simulink model "main_sim_adapt_Gref_SPPH"  (Simulink 7.2)
settings: Solver=ode2  SolverMode=SingleTasking  StartTime=0.0  StopTime=tsim_max  FixedStep=dtsim  RelTol=1e-3
StopFcn:
  | %mkplt
values from neighbouring files (symbols this model uses):
  assertion_time = inf    [setup_taem_sgs_al.m]
  cosA = cos(rwyAZ_rad)    [setup_taem_sgs_al.m]
  E_rwy = E_origin + (mod(( rwyLLA(2)/constants.r2d - lon_origin )+pi,2*pi)-pi) * constants.earth_radius * cos(lat_origin)    [setup_taem_sgs_al.m]
  eow_boundary = tmp_eow(ix(1))    [setup_taem_sgs_al.m]
  N_rwy = N_origin + (mod(( rwyLLA(1)/constants.r2d - lat_origin )+pi,2*pi)-pi) * constants.earth_radius    [setup_taem_sgs_al.m]
  sinA = sin(rwyAZ_rad)    [setup_taem_sgs_al.m]
  vel = 487.2512    [doit.m]
undefined symbols (not defined in the file or in its folder): accel_cmd, aero_surf_qbar_off, aero_surf_qbar_on, Alon, att_cmd_select, att_trim_IC, att_type, att_type_numbers, B1, bb_ellipsoid, bb_params, Blon, C, CA, chi_trim_IC, Clon, command_time, compute_all_rate_cols, compute_all_vel_cols, constants, da_trim_IC, dc_L2W_IC, de_trim_IC, DiscIntNeverNeededParam, dr_trim_IC, dtsim, DZkx, DZtheta, E_trim_IC, Ed_cmd, Ed_trim_IC, fc, flag_uad, full_surf_llim, full_surf_ulim, gain_set, gain_var_struct, gam_cmd_descent, gam_cmd_preflare, gamdot_cmd_descent, gamdot_cmd_flare, gamdot_cmd_preflare, gamma_trim_IC, Gamtheta, Gamx, h_trim_IC, hd_cmd, hd_trim_IC, ideal_vel_Kb, in_exsig_vecin, in_exsig_vecout, invCB, Kb, Kxhat0, Kxnom, Kxstar, lonxm0, MACH, MACH_att_fb, MACH_att_int_IC ... (+77)
libraries: simulink x36, utility_lib x36, mach_lib x24, model_lib x15, simulink_need_slupdate x8, models x6
(part 7 of 7)

== system main_sim_adapt_Gref_SPPH/claw_main/vel_loops/B matrix comp/B matrix comp/pert_comp ==
  col : Inport  OutDataType=sfix(16)  OutScaling=2^0
  d_nom : Inport  Port=2  OutDataType=sfix(16)  OutScaling=2^0
  params : Inport  Port=3  OutDataType=sfix(16)  OutScaling=2^0
  Bus Selector : BusSelector  OutputSignals=u_ulim,u_llim
  Constant2 : Constant  Value=diag(MACH.vel_u_pert)  OutDataType=sfix(16)  OutScaling=2^0
  pick +/- pert : mach_lib/pick +//- pert  SystemSampleTime=-1  num_u=MACH.vel_num_u
  d_pert : Outport  OutDataType=sfix(16)  OutScaling=2^0
  d_div : Outport  Port=2  OutDataType=sfix(16)  OutScaling=2^0
  wires:
  pick +/- pert/2 -> d_div/1  "scalar pert value"
  d_nom/1 -> pick +/- pert/2
  pick +/- pert/1 -> d_pert/1
  col/1 -> pick +/- pert/1
  Constant2/1 -> pick +/- pert/5
  params/1 -> Bus Selector/1
  Bus Selector/1 -> pick +/- pert/3  "<u_ulim>"
  Bus Selector/2 -> pick +/- pert/4  "<u_llim>"

== system main_sim_adapt_Gref_SPPH/claw_main/vel_loops/convert accel_cmd to NED_dd_cmd/vchigam_dot cmd/polar to cart ==
  note: Note: these are actually Vground and Vslant
  scaling_info : Inport  OutDataType=sfix(16)  OutScaling=2^0
  vchigam_dot_cmd : Inport  Port=2  OutDataType=sfix(16)  OutScaling=2^0
  Bus Selector : BusSelector  OutputSignals=Rground,Rslant
  Demux : Demux  Outputs=[1 2]
  Gain1 : Gain  Gain=[1 -1]  ParameterDataType=sfix(16)  ParameterScaling=2^0  OutDataType=sfix(16)  OutScaling=2^0
  Mux : Mux  Inputs=2
  Mux1 : Mux  Inputs=2
  Product3 : Product  OutDataType=sfix(16)  OutScaling=2^0  RndMeth=Zero
  along_dd;cross_dd;vert_dd : Outport  OutDataType=sfix(16)  OutScaling=2^0
  wires:
  scaling_info/1 -> Bus Selector/1
  Mux/1 -> Gain1/1
  vchigam_dot_cmd/1 -> Demux/1
  Bus Selector/1 -> Mux/1  "<Rground>"
  Bus Selector/2 -> Mux/2  "<Rslant>"
  Gain1/1 -> Product3/2
  Demux/2 -> Product3/1
  Demux/1 -> Mux1/1
  Product3/1 -> Mux1/2
  Mux1/1 -> along_dd;cross_dd;vert_dd/1

== system main_sim_adapt_Gref_SPPH/control input (modified)/control input/form control input/select command/att cmd select ==
  cmd_bus : Inport  OutDataType=sfix(16)  OutScaling=2^0
  Bus Selector1 : BusSelector  OutputSignals=att1_cmd,att2_cmd,att3_cmd,throttle_cmd  OutputAsBus=on
  Bus Selector2 : BusSelector  OutputSignals=att_cmd
  Switch : Switch  Threshold=0.5
  use_cam_rate_cmd1 : Constant  Value=att_cmd_select  OutDataType=sfix(16)  OutScaling=2^0
  att_cmd : Outport  OutDataType=sfix(16)  OutScaling=2^0
  wires:
  Switch/1 -> att_cmd/1
  use_cam_rate_cmd1/1 -> Switch/2
  cmd_bus/1 -> Bus Selector2/1, Bus Selector1/1
  Bus Selector2/1 -> Switch/1  "<att_cmd>"
  Bus Selector1/1 -> Switch/3

== system main_sim_adapt_Gref_SPPH/control input (modified)/control input/form control input/select command/pos cmd select ==
  cmd_bus : Inport  OutDataType=sfix(16)  OutScaling=2^0
  Bus Selector1 : BusSelector  OutputSignals=N_cmd,E_cmd,att3_cmd,h_cmd  OutputAsBus=on
  Bus Selector3 : BusSelector  OutputSignals=pos_cmd,accel_submode
  Bus Selector5 : BusSelector  OutputSignals=Vd_cmd,chid_cmd,att3_cmd,gammad_cmd  OutputAsBus=on
  Bus Selector6 : BusSelector  OutputSignals=Ndd_cmd,Edd_cmd,att3_cmd,hdd_cmd  OutputAsBus=on
  Constant : Constant  Value=use_NdEdh_pos  OutDataType=sfix(16)  OutScaling=2^0
  Ground : Ground
  Multiport Switch : MultiPortSwitch  Inputs=2  zeroidx=on
  Multiport Switch1 : MultiPortSwitch  Inputs=4  zeroidx=on
  Switch : Switch  Threshold=0.5
  convert if use_Vchigam : Subsystem
  use_cam_rate_cmd1 : Constant  Value=pos_cmd_select  OutDataType=sfix(16)  OutScaling=2^0
  pos_cmd : Outport  OutDataType=sfix(16)  OutScaling=2^0
  wires:
  Multiport Switch1/1 -> Switch/3
  Bus Selector5/1 -> Multiport Switch1/4
  Bus Selector6/1 -> Multiport Switch1/3
  Ground/1 -> Multiport Switch1/5
  Multiport Switch/1 -> Multiport Switch1/2
  Bus Selector3/2 -> Multiport Switch1/1  "<accel_submode>"
  Bus Selector3/1 -> Switch/1  "<pos_cmd>"
  Switch/1 -> pos_cmd/1
  use_cam_rate_cmd1/1 -> Switch/2
  cmd_bus/1 -> Bus Selector3/1, convert if use_Vchigam/1(cmd_bus), Bus Selector5/1, Bus Selector6/1, Bus Selector1/1
  Bus Selector1/1 -> Multiport Switch/2
  convert if use_Vchigam/1(pos_cmd) -> Multiport Switch/3
  Constant/1 -> Multiport Switch/1

== system main_sim_adapt_Gref_SPPH/control input (modified)/control input/form control input/select command/rate cmd select ==
  cmd_bus : Inport  OutDataType=sfix(16)  OutScaling=2^0
  Bus Selector1 : BusSelector  OutputSignals=p_cmd,q_cmd,r_cmd,throttle_cmd  OutputAsBus=on
  Bus Selector3 : BusSelector  OutputSignals=rate_cmd  OutputAsBus=on
  Switch : Switch  Threshold=0.5
  use_cam_rate_cmd1 : Constant  Value=rate_cmd_select  OutDataType=sfix(16)  OutScaling=2^0
  rate_cmd : Outport  OutDataType=sfix(16)  OutScaling=2^0
  wires:
  Bus Selector1/1 -> Switch/3
  Bus Selector3/1 -> Switch/1
  cmd_bus/1 -> Bus Selector1/1, Bus Selector3/1
  use_cam_rate_cmd1/1 -> Switch/2
  Switch/1 -> rate_cmd/1

== system main_sim_adapt_Gref_SPPH/control input (modified)/control input/form control input/select command/vel cmd select ==
  cmd_bus : Inport  OutDataType=sfix(16)  OutScaling=2^0
  Bus Selector1 : BusSelector  OutputSignals=Vd_cmd,chid_cmd,att3_cmd,gammad_cmd  OutputAsBus=on
  Bus Selector2 : BusSelector  OutputSignals=vel_cmd,accel_submode
  Bus Selector4 : BusSelector  OutputSignals=Ndd_cmd,Edd_cmd,att3_cmd,hdd_cmd  OutputAsBus=on
  Ground : Ground
  Multiport Switch : MultiPortSwitch  Inputs=4  zeroidx=on
  Switch : Switch  Threshold=0.5
  convert if use_Vchigam : Subsystem
  use_cam_rate_cmd1 : Constant  Value=vel_cmd_select  OutDataType=sfix(16)  OutScaling=2^0
  vel_cmd : Outport  OutDataType=sfix(16)  OutScaling=2^0
  wires:
  convert if use_Vchigam/1(vel_cmd) -> Multiport Switch/2
  Multiport Switch/1 -> Switch/3
  Bus Selector1/1 -> Multiport Switch/4
  Ground/1 -> Multiport Switch/5
  Bus Selector4/1 -> Multiport Switch/3
  Bus Selector2/2 -> Multiport Switch/1  "<accel_submode>"
  Bus Selector2/1 -> Switch/1  "<vel_cmd>"
  cmd_bus/1 -> convert if use_Vchigam/1(cmd_bus), Bus Selector1/1, Bus Selector4/1, Bus Selector2/1
  use_cam_rate_cmd1/1 -> Switch/2
  Switch/1 -> vel_cmd/1

== system main_sim_adapt_Gref_SPPH/control input (modified)/control input/generate commands/pos cmd generator/circle pos cmd ==
  cmd_bus : Inport  OutDataType=sfix(16)  OutScaling=2^0
  Bus Selector1 : BusSelector  OutputSignals=att3_cmd,h_cmd  OutputAsBus=on
  Constant : Constant  OutDataType=sfix(16)  OutScaling=2^0
  Gain : Gain  Gain=50  ParameterDataType=sfix(16)  ParameterScaling=2^0  OutDataType=sfix(16)  OutScaling=2^0
  Gain1 : Gain  Gain=50  ParameterDataType=sfix(16)  ParameterScaling=2^0  OutDataType=sfix(16)  OutScaling=2^0
  Gain2 : Gain  Gain=0.1  ParameterDataType=sfix(16)  ParameterScaling=2^0  OutDataType=sfix(16)  OutScaling=2^0
  Gain3 : Gain  ParameterDataType=sfix(16)  ParameterScaling=2^0  OutDataType=sfix(16)  OutScaling=2^0
  Mux1 : Mux  Inputs=3
  Ramp : Subsystem  mask{slope=1, start_time=command_time, initial_output=0, sample_time=MACH.dt}
      mask prompts: start_time "Start time:"; initial_output "Initial output:"; sample_time "Sample time (-1 for inherited):"
  Saturation1 : Saturate  UpperLimit=10  LowerLimit=0
  Sum : Sum  Inputs=|-+  OutDataType=sfix(16)  OutScaling=2^0
  Sum1 : Sum  Inputs=++|  OutDataType=sfix(16)  OutScaling=2^0
  Sum2 : Sum  Inputs=-+|  OutDataType=sfix(16)  OutScaling=2^0
  Trigonometric Function : Trigonometry
  Trigonometric Function1 : Trigonometry  Operator=cos
  pos_cmd : Outport  OutDataType=sfix(16)  OutScaling=2^0
  wires:
  Mux1/1 -> pos_cmd/1
  Bus Selector1/1 -> Mux1/3
  cmd_bus/1 -> Bus Selector1/1
  Gain3/1 -> Sum1/1
  Gain2/1 -> Trigonometric Function1/1, Trigonometric Function/1
  Saturation1/1 -> Gain3/1, Sum2/1
  Ramp/1(ramp) -> Sum2/2, Saturation1/1
  Gain/1 -> Sum1/2
  Sum1/1 -> Mux1/1
  Gain1/1 -> Mux1/2
  Constant/1 -> Sum/2
  Trigonometric Function1/1 -> Sum/1
  Sum2/1 -> Gain2/1
  Trigonometric Function/1 -> Gain/1
  Sum/1 -> Gain1/1

== system main_sim_adapt_Gref_SPPH/control input (modified)/control input/generate commands/pos cmd generator/ramp pos cmd ==
  cmd_bus : Inport  OutDataType=sfix(16)  OutScaling=2^0
  Bus Selector1 : BusSelector  OutputSignals=E_cmd,att3_cmd,h_cmd  OutputAsBus=on
  Discrete-Time Integrator1 : DiscreteIntegrator  SampleTime=-1  OutDataType=sfix(16)  OutScaling=2^0  ICPrevOutput=DiscIntNeverNeededParam  ICPrevScaledInput=DiscIntNeverNeededParam
  Discrete-Time Integrator3 : DiscreteIntegrator  SampleTime=-1  OutDataType=sfix(16)  OutScaling=2^0  ICPrevOutput=DiscIntNeverNeededParam  ICPrevScaledInput=DiscIntNeverNeededParam
  Gain : Gain  Gain=ideal_vel_Kb  ParameterDataType=sfix(16)  ParameterScaling=2^0  OutDataType=sfix(16)  OutScaling=2^0
  Mux : Mux  Inputs=2
  Sum6 : Sum  Inputs=|+-  OutDataType=sfix(16)  OutScaling=2^0  SaturateOnIntegerOverflow=on
  limit acceleration to g/3 : Saturate  UpperLimit=constants.g/3  LowerLimit=-constants.g/3
  velocity command : Step  Time=command_time  After=1.69*15  SampleTime=MACH.dt
  pos_cmd : Outport  OutDataType=sfix(16)  OutScaling=2^0
  wires:
  Bus Selector1/1 -> Mux/2
  cmd_bus/1 -> Bus Selector1/1
  Mux/1 -> pos_cmd/1
  Discrete-Time Integrator1/1 -> Mux/1
  Discrete-Time Integrator3/1 -> Sum6/2, Discrete-Time Integrator1/1
  velocity command/1 -> Sum6/1
  Sum6/1 -> Gain/1
  Gain/1 -> limit acceleration to g/3/1
  limit acceleration to g/3/1 -> Discrete-Time Integrator3/1

== system main_sim_adapt_Gref_SPPH/control input (modified)/control input/generate commands/vel cmd generator/Ramp ==
  From Workspace1 : FromWorkspace  VariableName=[ 0 initial_output ; start_time initial_output ; start_time+1 initial_output+slope ]  SampleTime=MACH.dt
  ramp : Outport  OutDataType=sfix(16)  OutScaling=2^0
  wires:
  From Workspace1/1 -> ramp/1

== system main_sim_adapt_Gref_SPPH/control input (modified)/control input/generate commands/vel cmd generator/descent ==
  From Workspace1 : FromWorkspace  VariableName=[ 0 initial_output ; start_time initial_output ; start_time+1 initial_output+slope ]  SampleTime=MACH.dt
  ramp : Outport  OutDataType=sfix(16)  OutScaling=2^0
  wires:
  From Workspace1/1 -> ramp/1

== system main_sim_adapt_Gref_SPPH/control input (modified)/control input/generate commands/vel cmd generator/flare ==
  From Workspace1 : FromWorkspace  VariableName=[ 0 initial_output ; start_time initial_output ; start_time+1 initial_output+slope ]  SampleTime=MACH.dt
  ramp : Outport  OutDataType=sfix(16)  OutScaling=2^0
  wires:
  From Workspace1/1 -> ramp/1

== system main_sim_adapt_Gref_SPPH/control input (modified)/control input/generate commands/vel cmd generator/pre-flare ==
  From Workspace1 : FromWorkspace  VariableName=[ 0 initial_output ; start_time initial_output ; start_time+1 initial_output+slope ]  SampleTime=MACH.dt
  ramp : Outport  OutDataType=sfix(16)  OutScaling=2^0
  wires:
  From Workspace1/1 -> ramp/1

== system main_sim_adapt_Gref_SPPH/control input (modified)/control input/generate commands/vel cmd generator/turn rate ==
  From Workspace1 : FromWorkspace  VariableName=[ 0 initial_output ; start_time initial_output ; start_time+1 initial_output+slope ]  SampleTime=MACH.dt
  ramp : Outport  OutDataType=sfix(16)  OutScaling=2^0
  wires:
  From Workspace1/1 -> ramp/1

== system main_sim_adapt_Gref_SPPH/control input (modified)/ideal responses/ideal att rate response/get att cmd/convert to quat ==
  att_cmd : Inport  OutDataType=sfix(16)  OutScaling=2^0
  e : Inport  Port=2  OutDataType=sfix(16)  OutScaling=2^0
  Demux : Demux  Outputs=[2 1]
  Discrete-Time Integrator4 : DiscreteIntegrator  IntegratorMethod=Integration: Backward Euler  InitialCondition=att_trim_IC(3)  SampleTime=-1  OutDataType=sfix(16)  OutScaling=2^0  ICPrevOutput=DiscIntNeverNeededParam  ICPrevScaledInput=DiscIntNeverNeededParam
  From Workspace2 : FromWorkspace  VariableName=use_cam_rate_cmd_fw  SampleTime=MACH.dt  Interpolate=off  OutputAfterFinalValue=Holding final value
  Multiport Switch1 : MultiPortSwitch  Inputs=2  zeroidx=on
  Mux2 : Mux  Inputs=2
  Selector : Selector  InputPortWidth=4  IndexOptions=Index vector (dialog)  Indices=[1 2 3]  OutputSizes=1
  att2dc : utility_lib/att2dc  SystemSampleTime=-1
  dc2e_ref : utility_lib/dc2e_ref  SystemSampleTime=-1
  e_cmd : Outport  OutDataType=sfix(16)  OutScaling=2^0
  wires:
  dc2e_ref/1 -> e_cmd/1
  Mux2/1 -> att2dc/1
  e/1 -> dc2e_ref/2
  att2dc/1 -> dc2e_ref/1
  Selector/1 -> Demux/1
  att_cmd/1 -> Selector/1
  Demux/1 -> Mux2/1
  Multiport Switch1/1 -> Mux2/2
  Demux/2 -> Discrete-Time Integrator4/1, Multiport Switch1/2
  Discrete-Time Integrator4/1 -> Multiport Switch1/3
  From Workspace2/1 -> Multiport Switch1/1

== system main_sim_adapt_Gref_SPPH/control input (modified)/control input/form control input/select command/pos cmd select/convert if use_Vchigam ==
  cmd_bus : Inport  OutDataType=sfix(16)  OutScaling=2^0
  Bus Assignment : BusAssignment  AssignedSignals=Nd_cmd,Ed_cmd
  Bus Selector3 : BusSelector  OutputSignals=Nd_cmd,Ed_cmd,att3_cmd,h_cmd  OutputAsBus=on
  Bus Selector5 : BusSelector  OutputSignals=V_cmd,chi_cmd,use_Vchigam
  Constant : Constant  Value=0  OutDataType=sfix(16)  OutScaling=2^0
  Switch : Switch  Threshold=0.5
  Terminator : Terminator
  vchigam2NdEdhd : utility_lib/vchigam2NdEdhd  SystemSampleTime=-1
  pos_cmd : Outport  OutDataType=sfix(16)  OutScaling=2^0
  wires:
  Constant/1 -> vchigam2NdEdhd/3
  Bus Selector5/2 -> vchigam2NdEdhd/2  "<chi_cmd>"
  Switch/1 -> pos_cmd/1
  Bus Assignment/1 -> Switch/1
  Bus Selector5/3 -> Switch/2  "<use_Vchigam>"
  Bus Selector3/1 -> Switch/3, Bus Assignment/1
  Bus Selector5/1 -> vchigam2NdEdhd/1  "<V_cmd>"
  vchigam2NdEdhd/3 -> Terminator/1
  vchigam2NdEdhd/2 -> Bus Assignment/3
  vchigam2NdEdhd/1 -> Bus Assignment/2
  cmd_bus/1 -> Bus Selector3/1, Bus Selector5/1

== system main_sim_adapt_Gref_SPPH/control input (modified)/control input/form control input/select command/vel cmd select/convert if use_Vchigam ==
  cmd_bus : Inport  OutDataType=sfix(16)  OutScaling=2^0
  Bus Assignment : BusAssignment  AssignedSignals=Nd_cmd,Ed_cmd,hd_cmd
  Bus Selector3 : BusSelector  OutputSignals=Nd_cmd,Ed_cmd,att3_cmd,hd_cmd  OutputAsBus=on
  Bus Selector5 : BusSelector  OutputSignals=V_cmd,chi_cmd,gamma_cmd,use_Vchigam
  Switch : Switch  Threshold=0.5
  vchigam2NdEdhd : utility_lib/vchigam2NdEdhd  SystemSampleTime=-1
  vel_cmd : Outport  OutDataType=sfix(16)  OutScaling=2^0
  wires:
  Switch/1 -> vel_cmd/1
  Bus Assignment/1 -> Switch/1
  Bus Selector5/4 -> Switch/2  "<use_Vchigam>"
  Bus Selector3/1 -> Switch/3, Bus Assignment/1
  Bus Selector5/3 -> vchigam2NdEdhd/3  "<gamma_cmd>"
  Bus Selector5/2 -> vchigam2NdEdhd/2  "<chi_cmd>"
  Bus Selector5/1 -> vchigam2NdEdhd/1  "<V_cmd>"
  vchigam2NdEdhd/3 -> Bus Assignment/4
  vchigam2NdEdhd/2 -> Bus Assignment/3
  vchigam2NdEdhd/1 -> Bus Assignment/2
  cmd_bus/1 -> Bus Selector3/1, Bus Selector5/1

== system main_sim_adapt_Gref_SPPH/control input (modified)/control input/generate commands/pos cmd generator/circle pos cmd/Ramp ==
  From Workspace1 : FromWorkspace  VariableName=[ 0 initial_output ; start_time initial_output ; start_time+1 initial_output+slope ]  SampleTime=MACH.dt
  ramp : Outport  OutDataType=sfix(16)  OutScaling=2^0
  wires:
  From Workspace1/1 -> ramp/1

== matlab function claw_main/rate_loops/allocation/RCS allocation/Embedded MATLAB Function ==
  data: Bmat input double; wght_cv input double; ulim input double; llim input double; cvd_des input double; rcs_cmd output double; minerr output double; scale output double; cvd_actual output double; err_thresh input double; rcs_use_in input double
function [rcs_cmd, minerr, scale, cvd_actual] = rcs_alloc(Bmat, wght_cv, ulim, llim, cvd_des, err_thresh, rcs_use_in)

rcs_quant = 0;
scale = 1;

nrcs = size(Bmat,2);


if(nrcs == 6)
    % assume fake RCS
    gang_pos = [0 0 0; 0 0 0; 1 1 0; 1 0 0; 0 0 1; 0 1 0];
    gang_neg = [1 1 0; 0 0 1; 0 0 0; 0 1 0; 0 0 0; 1 0 0];

    gain_factor = 1./diag(Bmat*gang_pos);
    rcs_cmd = gang_neg*(gain_factor.*max(0,-cvd_des)) + gang_pos*(gain_factor.*max(0,cvd_des));
    if(rcs_quant > 0)
        rcs_cmd = round(rcs_cmd/rcs_quant)*rcs_quant;
    end
    rcs_cmd = max(min(rcs_cmd,ulim),llim);
    cvd_actual = Bmat*rcs_cmd;
    minerr = norm_vec(cvd_actual - cvd_des);
    
    return
end

rcs_cmd = llim;
cvd_actual = Bmat*rcs_cmd; 
minerr = norm_vec((cvd_actual - cvd_des).*wght_cv);

if(minerr <= err_thresh)
    return
end

Bmat = diag(wght_cv)*Bmat;
cvd_des = wght_cv.*cvd_des;

scale_trial = 1;
normsq_cvd_trial = 0;

powersof2 = 2.^[0:nrcs-1];
bllim = uint32(powersof2*llim);
bulim = uint32(powersof2*ulim);
rcs_use_all = uint32([1:2^nrcs-1]');
rcs_use_tmp = bitor(rcs_use_all,uint32(bllim));
rcs_use_tmp = bitand(rcs_use_tmp,uint32(bulim));
rcs_use = rcs_use_in.*eq(rcs_use_tmp,rcs_use_all);

if(~any(rcs_use))
    return
end

for i = 1:length(rcs_use)
    
    if(~rcs_use(i))
        continue
    end
    
    rcson = double(bitget(uint32(i),1:nrcs))';
    cvd_trial = Bmat*rcson;
    
    % optional scaling
    if(0)
        scale_trial = dot(cvd_des,cvd_trial);
        if(scale_trial < 0)
            continue
        end
        
        normsq_cvd_trial = dot(cvd_trial,cvd_trial);
        if(normsq_cvd_trial <= scale_trial)
            scale_trial = 1;
        else
            scale_trial = dot(cvd_des,cvd_trial)/normsq_cvd_trial;
            cvd_trial = cvd_trial*scale_trial;
        end
    end
    
    cvd_ex = cvd_trial - cvd_des;
    err = norm_vec(cvd_ex);
    if(err < minerr)
        scale = scale_trial;
        rcs_cmd = rcson*scale;
        minerr = err;
        cvd_actual = cvd_trial./wght_cv;
    end
end

function out = norm_vec(in)

out = sqrt(sum(in.^2));

return

== matlab function claw_main/rate_loops/bangbang/Bang Bang ==
  data: bb_params input double; bb_ellipsoid input double; debug_output output double; cvddes output double; dir output double; use_bb output double; att_cvc input double; att_cv input double; timer output double; pqr input double; inertia input double; enable_bb input double; cvddes_lin input double; dir_old input double; use_bb_old input double; timer_old input double
function [debug_output,cvddes,dir,use_bb,timer] = bangbang(bb_params,bb_ellipsoid,att_cvc,att_cv,pqr,inertia,enable_bb,cvddes_lin,dir_old,use_bb_old,timer_old)
% This block supports an embeddable subset of the MATLAB language.
% See the help menu for details. 

dt = bb_params(1) ;
timer_max = bb_params(2) ;
att_thresh = bb_params(3) ;
rate_thresh = bb_params(4) ;
att_diff_thresh = bb_params(5) ;
pp_params = bb_params(6:end) ;

debug_output = zeros(12,1) ;
cvddes = cvddes_lin ;
use_bb = 0 ;
dir = zeros(3,1) ;
timer = timer_old ;

if( ~enable_bb )
    return
end
    
trans = qmpy([1 -1 -1 -1]'.*att_cv,att_cvc) ;

% default is to use dir_old if we were in bangbang last cycle,
% and the timer has not expired
use_dir_old = use_bb_old ;
if( use_dir_old )
    timer = timer + dt ;
    if( timer > timer_max )
        % if timer expires, don't use dir_old
        use_dir_old = 0 ;
    end
end

% compute att using current transformation quat
trans_mag = trans(1) ;
trans_dir = trans(2:4) ;
att = -2*atan2(norm_vec3(trans_dir),trans_mag) ;
att_old = -2*atan2(dir_old'*trans_dir,trans_mag) ;

% choose arbitrary att (and dir) sign to be the same as that computed using
% dir_old.  This is equivalent to making dir_old'*trans_dir positive.
if( att*att_old < 0 )
    att = -att ;
    trans_dir = -trans_dir ;
end

% if we intended to use dir_old, but the angle computed using
% dir_old is significantly different than that derived using the current
% transformation, we will use current dir.
% NOTE: the angle test below works only because att has been adjusted
% to have the same sign as att_old, and both result from atan2 
if( use_dir_old )
    if( abs(att - att_old) > att_diff_thresh )
        use_dir_old = 0 ;
    else
        dir = dir_old ;
        att = att_old ;
    end
end

% check condition to enter (or stay in) bangbang
if( abs(att) > att_thresh )
    use_bb = 1 ;
    
    if( ~use_dir_old )
        dir = trans_dir/norm_vec3(trans_dir) ;
        timer = 0 ;
    end

elseif( max(abs(pqr)) > rate_thresh )
    use_bb = 1 ;
    
    % if small attitude error, set dir based on rates
    if( ~use_dir_old )
        dir = pqr/norm_vec3(pqr) ;
        att = -2*atan2(dir'*trans_dir,trans_mag) ;
        timer = 0 ;
    end
else
    % even though not used, pass dir_old through for in case of ~use_bb
    dir = dir_old ;
    att = att_old ;
end

% Note: cvddes has been set to a default value of cvddes_lin

if( use_bb )
    rate = pqr'*dir ;
    accel_max = get_ellipsoid_scaling(inertia*dir,bb_ellipsoid) ;
    accel_min = -accel_max ;
    pp_params(1) = accel_max ;
    pp_params(2) = accel_min ;
    [outside,accel] = pp(pp_params,att,rate) ;
    
    if( outside <= 1 )
        % use default cvddes (cvddes_lin)
        use_bb = 0 ; 
    else
        % eliminate component of linear command in direction dir
        cvddes = cvddes - (dir'*cvddes)*dir ;
    end
else
    % use default cvddes (cvddes_lin)
    rate = 0 ;
    outside = 0 ;
    accel = 0 ;
end

% saturate command at ellipsoid
blend_lin_claw = cvddes*min(get_ellipsoid_scaling(inertia*cvddes,bb_ellipsoid),1) ;

% add component from bangbang
blend_bb_claw = accel*dir ;
cvddes = blend_lin_claw + blend_bb_claw ;

pp_utQu = 1/get_ellipsoid_scaling(inertia*cvddes,bb_ellipsoid) ;
debug_output = [att;att_old;rate;outside;accel;pp_utQu;blend_bb_claw;blend_lin_claw] ;

if( ~use_bb )
    
    % if not using bangbang reset the timer, and set dir to zero
    timer = 0 ;
    % dir used for cvd_des blending is now zeroed outside of this block,
    % so that dir can be retained through a temporary ~use_bb condition
%     dir = 0*dir ;
end

function r = qmpy(p,q)

p0 = p(1) ;
p1 = p(2) ;
p2 = p(3) ;
p3 = p(4) ;

q0 = q(1) ;
q1 = q(2) ;
q2 = q(3) ;
q3 = q(4) ;

r0 = p0 * q0 - p1 * q1 - p2 * q2 - p3 * q3 ;
r1 = p0 * q1 + p1 * q0 + p2 * q3 - p3 * q2 ;
r2 = p0 * q2 - p1 * q3 + p2 * q0 + p3 * q1 ;
r3 = p0 * q3 + p1 * q2 - p2 * q1 + p3 * q0 ;

r = [ r0 r1 r2 r3 ]' ;

function scale = get_ellipsoid_scaling(dir,ellipsoid)
    scale = 1/max(sqrt(dir'*(ellipsoid*dir)),1e-12) ;

function [outside,accel] = pp(params,att,rate)

% the linear control law is
% accel = ww^2 * ( att_cmd - att ) - 2 * zeta * ww * rate

amax = params(1) ; 
amin = params(2) ; 
ww = params(3) ;  
zeta = params(4) ; 
rate_des1 = params(5) ; 
rate_des2 = params(6) ;

% make switch curves conservative
swcurve_shrink = 1.0 ;

swcurve_pos = 0.5 * rate^2 - swcurve_shrink * amin * att ;
swcurve_neg = 0.5 * rate^2 - swcurve_shrink * amax * att ;

% replace ellipse with parallelogram
% outside = ( ww^2 * att^2 + 2 * zeta * ww * att * rate + rate^2 ) / ( ( 1 - zeta^2 ) * amax^2 / ww^2 ) ;
sx1 = 1 + zeta + 4 * zeta^2 ;
sv1 = -0.5 - 2 * zeta ;
sx2 = 1 - 4 * zeta^2
sv2 = 2 * zeta ;
p1 = [sx1; sv1] ;
p2 = [sx2; sv2] ;

outside = 2*ww/amax*max(abs(([p2+p1 p2-p1]\[att*ww; rate])))
accel = 0 ;

if( outside <= 1 )
    return
end

if( rate > 0 )
    if( swcurve_pos < 0 )
        if( rate < rate_des1 )
            accel = amax ;
        elseif( rate < rate_des2 )
            accel = 0 ;
        else
            accel = amin ;
        end
    else
        accel = amin ;
    end
else
    if( swcurve_neg < 0 )
        if( rate > -rate_des1 )
            accel = amin ;
        elseif( rate > - rate_des2 )
            accel = 0 ;
        else
            accel = amax ;
        end
    else
        accel = amax ;
    end
end


function out = norm_vec3(in)

out = sqrt(in(1)^2 + in(2)^2 + in(3)^2);

return
